simulink model "diffusionTest"  (R2022a)
settings: Solver=VariableStepAuto  StartTime=0.0  StopTime=10.0  RelTol=1e-3
settings Model: Creator=mateu  LastModifiedBy=mateu

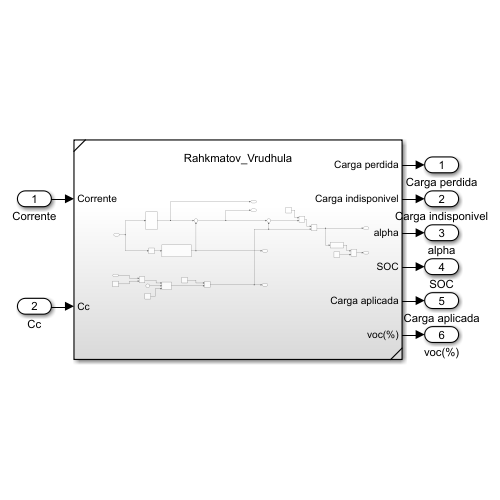
[thumbnail: Simulink's stored preview of the top-level diagram]
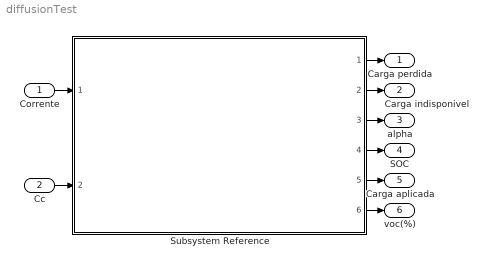
== system diffusionTest ==
  Corrente : Inport
  Cc : Inport  Port=2
  Subsystem Reference : Subsystem  ReferencedSubsystem=Rahkmatov_Vrudhula
  Carga perdida : Outport
  Carga indisponivel : Outport  Port=2
  alpha : Outport  Port=3
  SOC : Outport  Port=4
  Carga aplicada : Outport  Port=5
  voc(%) : Outport  Port=6
  wires:
  Cc/1 -> Subsystem Reference/2
  Subsystem Reference/1 -> Carga perdida/1
  Subsystem Reference/2 -> Carga indisponivel/1
  Corrente/1 -> Subsystem Reference/1
  Subsystem Reference/6 -> voc(%)/1
  Subsystem Reference/5 -> Carga aplicada/1
  Subsystem Reference/4 -> SOC/1
  Subsystem Reference/3 -> alpha/1
